simulink model "simple_car_model"  (R2017a)
settings: Solver=VariableStepAuto  StartTime=0.0  StopTime=10.0  RelTol=1e-3
undefined symbols (not defined in the file): k, m, v0, x0
settings Model: Creator=jyotirmoy  LastModifiedBy=jyotirmoy

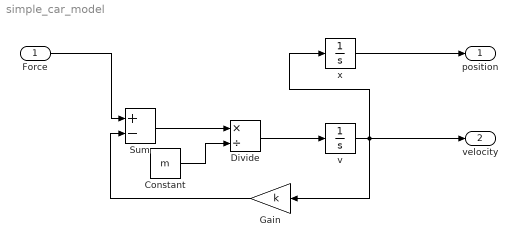
== system simple_car_model ==
  Force : Inport
  Constant : Constant  Value=m
  Divide : Product  Inputs=*/
  Gain : Gain  Gain=k
  Sum : Sum  Inputs=+-
  v : Integrator  InitialCondition=v0
  x : Integrator  InitialCondition=x0
  position : Outport
  velocity : Outport  Port=2
  wires:
  Force/1 -> Sum/1
  v/1 -> Gain/1, velocity/1, x/1
  Sum/1 -> Divide/1
  Gain/1 -> Sum/2
  x/1 -> position/1
  Divide/1 -> v/1
  Constant/1 -> Divide/2
